simulink model "OSWEC"
settings: Solver=ode4  StartTime=0  StopTime=400  FixedStep=0.1  RelTol=1e-3  EnableMultiTasking=on
undefined symbols (not defined in the file): body, constraint, pto
libraries: WECSim_Lib x5

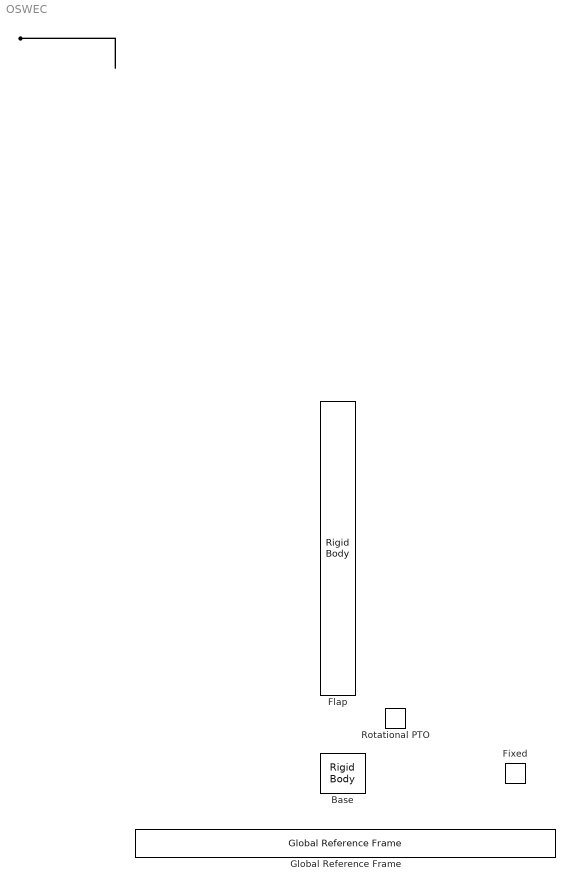
== system OSWEC ==
  Base : WECSim_Lib/Body Elements/Rigid Body  body=body(2)  body=body(2)  body=body(2)  body=body(2)
      settings: AttributesFormatString=%<body>
  Fixed : WECSim_Lib/Constraints/Fixed  constraint=constraint(1)  constraint=constraint(1)  constraint=constraint(1)  constraint=constraint(1)
      settings: AttributesFormatString=%<constraint>
  Flap : WECSim_Lib/Body Elements/Rigid Body  body=body(1)  body=body(1)  body=body(1)  body=body(1)
      settings: AttributesFormatString=%<body>
  Global Reference Frame : WECSim_Lib/Frames/Global Reference Frame  waves=waves  simu=simu  waves=waves  simu=simu  waves=waves  simu=simu  waves=waves  simu=simu
  Rotational PTO : WECSim_Lib/PTOs/Rotational PTO  pto=pto(1)  pto=pto(1)  pto=pto(1)  pto=pto(1)
      settings: AttributesFormatString=%<pto>
  connections:
  ?
  ?
  ?
